simulink model "Sliding"  (R2023a)
settings: Solver=VariableStepAuto  StartTime=0.0  StopTime=7.32  RelTol=1e-3
settings Model: Creator=HP  LastModifiedBy=28012
settings SolverCC: ZeroCrossAlgorithm=Adaptive  AlgebraicLoopSolver=TrustRegion
settings DataIOCC: ReturnWorkspaceOutputs=off
settings DebuggingCC: IgnoredZcDiagnostic=none  UnconnectedInputMsg=warning  UnconnectedOutputMsg=warning  UnconnectedLineMsg=warning  ArithmeticOperatorsInVariantConditions=warning
settings ModelReferenceCC: EnableRefExpFcnMdlSchedulingChecks=on
settings SFSimCC: SimUseLocalCustomCode=off  CustomCodeUndefinedFunction=UseInterfaceOnly
settings RTWCC: RTWUseLocalCustomCode=off

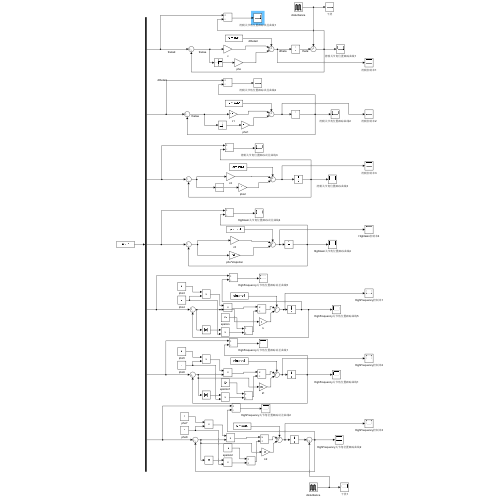
[thumbnail: Simulink's stored preview of the top-level diagram]
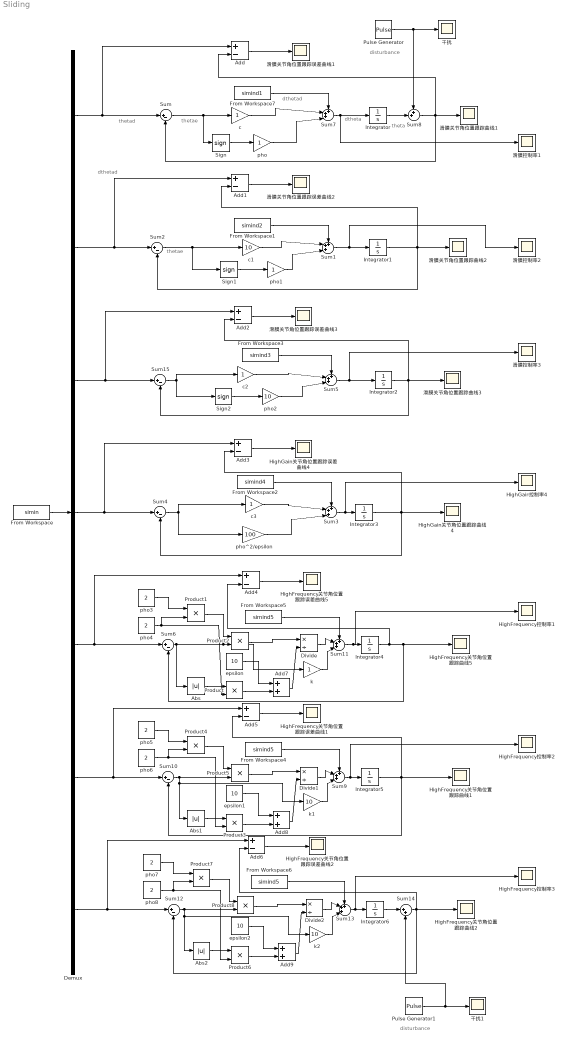
== system Sliding ==
  note: disturbance
  note: dtheta
  note: dthetad
  note: thetae
  note: thetad
  note: theta
  note: thetae
  note: dthetad
  note: disturbance
  Abs : Abs  SaturateOnIntegerOverflow=off
  Abs1 : Abs  SaturateOnIntegerOverflow=off
  Abs2 : Abs  SaturateOnIntegerOverflow=off
  Add{,1..6} (7 alike) : Sum  Inputs=+-
  Add7 : Sum
  Add8 : Sum
  Add9 : Sum
  Demux : Demux  Outputs=7
  Divide : Product  Inputs=*/
  Divide1 : Product  Inputs=*/
  Divide2 : Product  Inputs=*/
  From Workspace : FromWorkspace  VariableName=simin
  From Workspace1 : FromWorkspace  VariableName=simind2
  From Workspace2 : FromWorkspace  VariableName=simind4
  From Workspace3 : FromWorkspace  VariableName=simind3
  From Workspace4 : FromWorkspace  VariableName=simind5
  From Workspace5 : FromWorkspace  VariableName=simind5
  From Workspace6 : FromWorkspace  VariableName=simind5
  From Workspace7 : FromWorkspace  VariableName=simind1
  HighFrequency关节角位置跟踪曲线1 : Scope
  HighFrequency关节角位置跟踪曲线2 : Scope
  HighFrequency关节角位置跟踪曲线5 : Scope
  HighFrequency关节角位置跟踪误差曲线1 : Scope
  HighFrequency关节角位置跟踪误差曲线2 : Scope
  HighFrequency关节角位置跟踪误差曲线5 : Scope
  HighFrequency控制率1 : Scope
  HighFrequency控制率2 : Scope
  HighFrequency控制率3 : Scope
  HighGain关节角位置跟踪曲线4 : Scope
  HighGain关节角位置跟踪误差曲线4 : Scope
  HighGain控制率4 : Scope
  Integrator{,1..6} (7 alike) : Integrator  InitialCondition=1
  Product{,1..8} (9 alike) : Product
  Pulse Generator : DiscretePulseGenerator  PulseType=Time based  Amplitude=0.1  Period=1  PulseWidth=20  PhaseDelay=2
  Pulse Generator1 : DiscretePulseGenerator  PulseType=Time based  Amplitude=0.1  Period=1  PulseWidth=20  PhaseDelay=2
  Sign : Signum
  Sign1 : Signum
  Sign2 : Signum
  Sum : Sum  Inputs=|+-
  Sum{1,3,5,7,9,11,13} (7 alike) : Sum  Inputs=+++|  InputSameDT=on  SaturateOnIntegerOverflow=on  OutDataTypeStr=Inherit: Same as first input
  Sum{2,4,6,10,12,15} (6 alike) : Sum  Inputs=|+-  InputSameDT=on  SaturateOnIntegerOverflow=on  OutDataTypeStr=Inherit: Same as first input
  Sum14 : Sum  Inputs=|++  InputSameDT=on  SaturateOnIntegerOverflow=on  OutDataTypeStr=Inherit: Same as first input
  Sum8 : Sum  Inputs=++|
  c : Gain
  c1 : Gain  Gain=10
  c2 : Gain
  c3 : Gain
  epsilon : Constant  Value=10
  epsilon1 : Constant  Value=10
  epsilon2 : Constant  Value=10
  k : Gain
  k1 : Gain  Gain=10
  k2 : Gain  Gain=10
  pho : Gain
  pho1 : Gain
  pho2 : Gain  Gain=10
  pho{3..8} (6 alike) : Constant  Value=2
  pho^2/epsilon : Gain  Gain=100
  干扰 : Scope
  干扰1 : Scope
  滑膜关节角位置跟踪曲线1 : Scope
  滑膜关节角位置跟踪曲线2 : Scope
  滑膜关节角位置跟踪曲线3 : Scope
  滑膜关节角位置跟踪误差曲线1 : Scope
  滑膜关节角位置跟踪误差曲线2 : Scope
  滑膜关节角位置跟踪误差曲线3 : Scope
  滑膜控制率1 : Scope
  滑膜控制率2 : Scope
  滑膜控制率3 : Scope
  wires:
  Add/1 -> 滑膜关节角位置跟踪误差曲线1/1
  Sum7/1 -> 滑膜控制率1/1, Integrator/1
  From Workspace7/1 -> Sum7/1
  Demux/1 -> Sum/1, Add/1
  From Workspace1/1 -> Sum1/1
  Add1/1 -> 滑膜关节角位置跟踪误差曲线2/1
  Sum1/1 -> 滑膜控制率2/1, Integrator1/1
  From Workspace/1 -> Demux/1
  Demux/2 -> Sum2/1, Add1/1
  From Workspace3/1 -> Sum5/1
  Demux/3 -> Sum15/1, Add2/1
  Add2/1 -> 滑膜关节角位置跟踪误差曲线3/1
  Sum3/1 -> HighGain控制率4/1, Integrator3/1
  Add3/1 -> HighGain关节角位置跟踪误差曲线4/1
  Demux/4 -> Sum4/1, Add3/1
  Sum5/1 -> 滑膜控制率3/1, Integrator2/1
  Demux/5 -> Sum6/1, Add4/1
  Add4/1 -> HighFrequency关节角位置跟踪误差曲线5/1
  Sum11/1 -> HighFrequency控制率1/1, Integrator4/1
  Integrator/1 -> Sum8/2
  Pulse Generator/1 -> 干扰/1, Sum8/1
  Sum8/1 -> Sum/2, Add/2, 滑膜关节角位置跟踪曲线1/1
  Integrator1/1 -> Sum2/2, Add1/2, 滑膜关节角位置跟踪曲线2/1
  Integrator2/1 -> Sum15/2, Add2/2, 滑膜关节角位置跟踪曲线3/1
  Integrator3/1 -> Sum4/2, Add3/2, HighGain关节角位置跟踪曲线4/1
  From Workspace2/1 -> Sum3/1
  From Workspace5/1 -> Sum11/1
  Integrator4/1 -> HighFrequency关节角位置跟踪曲线5/1, Sum6/2, Add4/2
  Sum/1 -> Sign/1, c/1
  Sign/1 -> pho/1
  c/1 -> Sum7/2
  pho/1 -> Sum7/3
  Sign1/1 -> pho1/1
  Sum2/1 -> Sign1/1, c1/1
  c1/1 -> Sum1/2
  pho1/1 -> Sum1/3
  Sign2/1 -> pho2/1
  Sum15/1 -> Sign2/1, c2/1
  c2/1 -> Sum5/2
  pho2/1 -> Sum5/3
  Sum4/1 -> pho^2/epsilon/1, c3/1
  c3/1 -> Sum3/2
  pho^2/epsilon/1 -> Sum3/3
  Sum6/1 -> k/1, Product2/2, Abs/1
  pho3/1 -> Product1/1
  pho4/1 -> Product/2, Product1/2
  Abs/1 -> Product/1
  Product/1 -> Add7/2
  epsilon/1 -> Add7/1
  Product1/1 -> Product2/1
  Product2/1 -> Divide/1
  Add7/1 -> Divide/2
  Divide/1 -> Sum11/2
  k/1 -> Sum11/3
  Product3/1 -> Add8/2
  pho5/1 -> Product4/1
  k1/1 -> Sum9/3
  pho6/1 -> Product3/2, Product4/2
  Abs1/1 -> Product3/1
  Product4/1 -> Product5/1
  epsilon1/1 -> Add8/1
  Add8/1 -> Divide1/2
  Product5/1 -> Divide1/1
  Sum10/1 -> k1/1, Abs1/1, Product5/2
  Sum9/1 -> HighFrequency控制率2/1, Integrator5/1
  Integrator5/1 -> Add5/2, Sum10/2, HighFrequency关节角位置跟踪曲线1/1
  From Workspace4/1 -> Sum9/1
  Add5/1 -> HighFrequency关节角位置跟踪误差曲线1/1
  Demux/6 -> Sum10/1, Add5/1
  Divide1/1 -> Sum9/2
  Sum12/1 -> k2/1, Abs2/1, Product8/2
  Sum13/1 -> HighFrequency控制率3/1, Integrator6/1
  Divide2/1 -> Sum13/2
  Add6/1 -> HighFrequency关节角位置跟踪误差曲线2/1
  From Workspace6/1 -> Sum13/1
  Product8/1 -> Divide2/1
  Add9/1 -> Divide2/2
  epsilon2/1 -> Add9/1
  Product6/1 -> Add9/2
  Abs2/1 -> Product6/1
  Product7/1 -> Product8/1
  pho7/1 -> Product7/1
  pho8/1 -> Product6/2, Product7/2
  k2/1 -> Sum13/3
  Demux/7 -> Add6/1, Sum12/1
  Pulse Generator1/1 -> Sum14/2, 干扰1/1
  Integrator6/1 -> Sum14/1
  Sum14/1 -> Add6/2, Sum12/2, HighFrequency关节角位置跟踪曲线2/1
